simulink model "LUTs"  (Simulink 5.0)
settings: Solver=ode45  StartTime=0.0  StopTime=10.0  RelTol=1e-3
undefined symbols (not defined in the file or in its folder): a_vec, b, Cbar, h_vec, J_FDIR, p_vec, r2d, rho_vec, S, splr_vec, T_vec, weight
libraries: simulink x14
settings Model: LastModifiedBy=Gpapageo

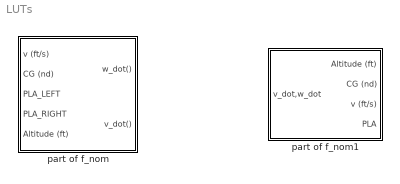
== system LUTs ==
  part of f_nom : Subsystem
  part of f_nom1 : Subsystem  Orientation=left

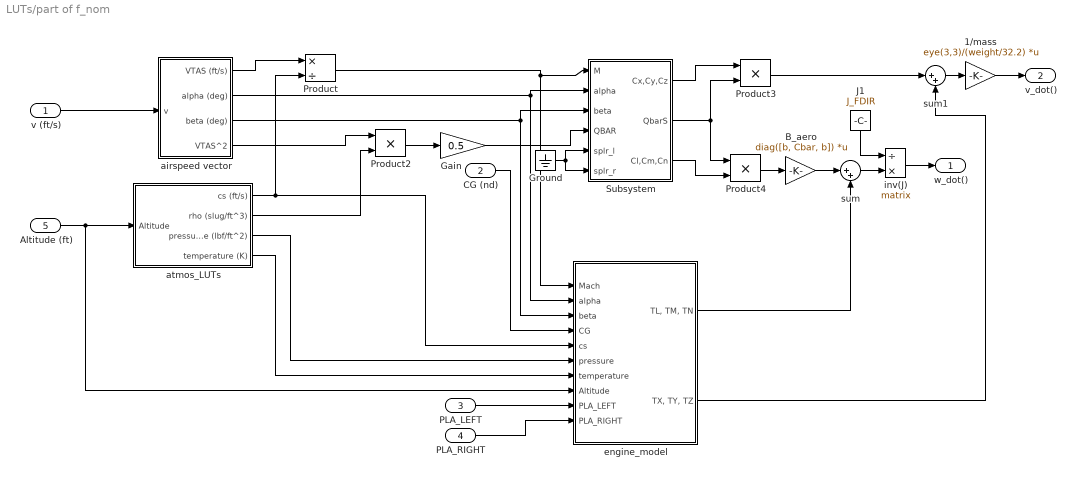
== system LUTs/part of f_nom ==
  v (ft/s) : Inport
  CG (nd) : Inport  Port=2
  PLA_LEFT : Inport  Port=3
  PLA_RIGHT : Inport  Port=4
  Altitude (ft) : Inport  Port=5
  1/mass : Gain  Gain=eye(3,3)/(weight/32.2)  Multiplication=Matrix(K*u)  SaturateOnIntegerOverflow=on
  B_aero : Gain  Gain=diag([b, Cbar, b])  Multiplication=Matrix(K*u)  SaturateOnIntegerOverflow=on
  Gain : Gain  Gain=0.5  SaturateOnIntegerOverflow=on
  Ground : Ground
  J1 : Constant  Orientation=down  Value=J_FDIR
  Product : Product  Inputs=*/  SaturateOnIntegerOverflow=on
  Product2 : Product  SaturateOnIntegerOverflow=on
  Product3 : Product  SaturateOnIntegerOverflow=on
  Product4 : Product  SaturateOnIntegerOverflow=on
  Subsystem : Subsystem
  airspeed vector : Subsystem
  atmos_LUTs : Subsystem
  engine_model : Subsystem
  inv(J) : Product  Inputs=/*  Multiplication=Matrix(*)  SaturateOnIntegerOverflow=on  InputSameDT=on
  sum : Sum  Inputs=|++  InputSameDT=on
  sum1 : Sum  Inputs=|++  InputSameDT=on
  w_dot() : Outport
  v_dot() : Outport  Port=2
  wires:
  sum1/1 -> 1/mass/1
  engine_model/1("TL, TM, TN") -> sum/2
  engine_model/2("TX, TY, TZ") -> sum1/2
  Product3/1 -> sum1/1
  1/mass/1 -> v_dot()/1
  sum/1 -> inv(J)/2
  B_aero/1 -> sum/1
  Subsystem/2(QbarS) -> Product4/1, Product3/2
  Subsystem/3(Cl,Cm,Cn) -> Product4/2
  Subsystem/1(Cx,Cy,Cz) -> Product3/1
  inv(J)/1 -> w_dot()/1
  Product4/1 -> B_aero/1
  J1/1 -> inv(J)/1
  PLA_RIGHT/1 -> engine_model/10(PLA_RIGHT)
  PLA_LEFT/1 -> engine_model/9(PLA_LEFT)
  atmos_LUTs/4(temperature (K)) -> engine_model/7(temperature)
  atmos_LUTs/3(pressure (lbf/ft^2)) -> engine_model/6(pressure)
  atmos_LUTs/1(cs (ft/s)) -> engine_model/5(cs), Product/2
  Product2/1 -> Gain/1
  airspeed vector/4(VTAS^2) -> Product2/1
  CG (nd)/1 -> engine_model/4(CG)
  v (ft/s)/1 -> airspeed vector/1(v)
  Altitude (ft)/1 -> engine_model/8(Altitude), atmos_LUTs/1(Altitude)
  atmos_LUTs/2(rho (slug/ft^3)) -> Product2/2
  airspeed vector/1(VTAS (ft/s)) -> Product/1
  airspeed vector/3(beta (deg)) -> engine_model/3(beta), Subsystem/3(beta)
  airspeed vector/2(alpha (deg)) -> engine_model/2(alpha), Subsystem/2(alpha)
  Product/1 -> engine_model/1(Mach), Subsystem/1(M)
  Gain/1 -> Subsystem/4(QBAR)
  Ground/1 -> Subsystem/5(splr_l), Subsystem/6(splr_r)

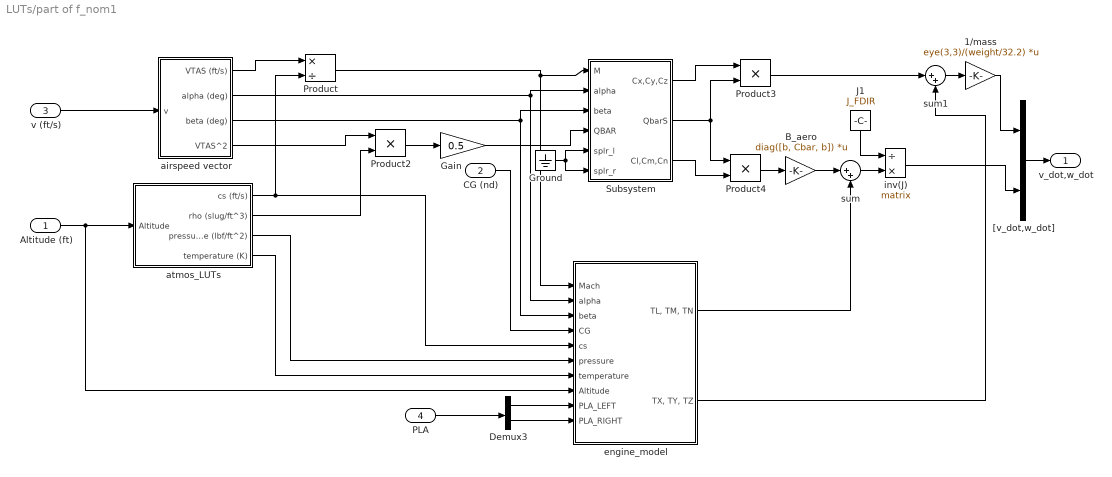
== system LUTs/part of f_nom1 ==
  Altitude (ft) : Inport
  CG (nd) : Inport  Port=2
  v (ft/s) : Inport  Port=3
  PLA : Inport  Port=4
  1/mass : Gain  Gain=eye(3,3)/(weight/32.2)  Multiplication=Matrix(K*u)  SaturateOnIntegerOverflow=on
  B_aero : Gain  Gain=diag([b, Cbar, b])  Multiplication=Matrix(K*u)  SaturateOnIntegerOverflow=on
  Demux3 : Demux  Outputs=2
  Gain : Gain  Gain=0.5  SaturateOnIntegerOverflow=on
  Ground : Ground
  J1 : Constant  Orientation=down  Value=J_FDIR
  Product : Product  Inputs=*/  SaturateOnIntegerOverflow=on
  Product2 : Product  SaturateOnIntegerOverflow=on
  Product3 : Product  SaturateOnIntegerOverflow=on
  Product4 : Product  SaturateOnIntegerOverflow=on
  Subsystem : Subsystem
  "[v_dot,w_dot]" : Mux  Inputs=[3 3]
  airspeed vector : Subsystem
  atmos_LUTs : Subsystem
  engine_model : Subsystem
  inv(J) : Product  Inputs=/*  Multiplication=Matrix(*)  SaturateOnIntegerOverflow=on  InputSameDT=on
  sum : Sum  Inputs=|++  InputSameDT=on
  sum1 : Sum  Inputs=|++  InputSameDT=on
  v_dot,w_dot : Outport
  wires:
  Ground/1 -> Subsystem/6(splr_r), Subsystem/5(splr_l)
  Gain/1 -> Subsystem/4(QBAR)
  Product/1 -> Subsystem/1(M), engine_model/1(Mach)
  airspeed vector/2(alpha (deg)) -> Subsystem/2(alpha), engine_model/2(alpha)
  airspeed vector/3(beta (deg)) -> Subsystem/3(beta), engine_model/3(beta)
  airspeed vector/1(VTAS (ft/s)) -> Product/1
  atmos_LUTs/2(rho (slug/ft^3)) -> Product2/2
  Altitude (ft)/1 -> atmos_LUTs/1(Altitude), engine_model/8(Altitude)
  v (ft/s)/1 -> airspeed vector/1(v)
  CG (nd)/1 -> engine_model/4(CG)
  airspeed vector/4(VTAS^2) -> Product2/1
  Product2/1 -> Gain/1
  atmos_LUTs/1(cs (ft/s)) -> Product/2, engine_model/5(cs)
  atmos_LUTs/3(pressure (lbf/ft^2)) -> engine_model/6(pressure)
  atmos_LUTs/4(temperature (K)) -> engine_model/7(temperature)
  J1/1 -> inv(J)/1
  Product4/1 -> B_aero/1
  Subsystem/1(Cx,Cy,Cz) -> Product3/1
  Subsystem/3(Cl,Cm,Cn) -> Product4/2
  Subsystem/2(QbarS) -> Product3/2, Product4/1
  B_aero/1 -> sum/1
  sum/1 -> inv(J)/2
  Product3/1 -> sum1/1
  engine_model/2("TX, TY, TZ") -> sum1/2
  engine_model/1("TL, TM, TN") -> sum/2
  sum1/1 -> 1/mass/1
  PLA/1 -> Demux3/1
  Demux3/1 -> engine_model/9(PLA_LEFT)
  Demux3/2 -> engine_model/10(PLA_RIGHT)
  inv(J)/1 -> "[v_dot,w_dot]"/2
  "[v_dot,w_dot]"/1 -> v_dot,w_dot/1
  1/mass/1 -> "[v_dot,w_dot]"/1

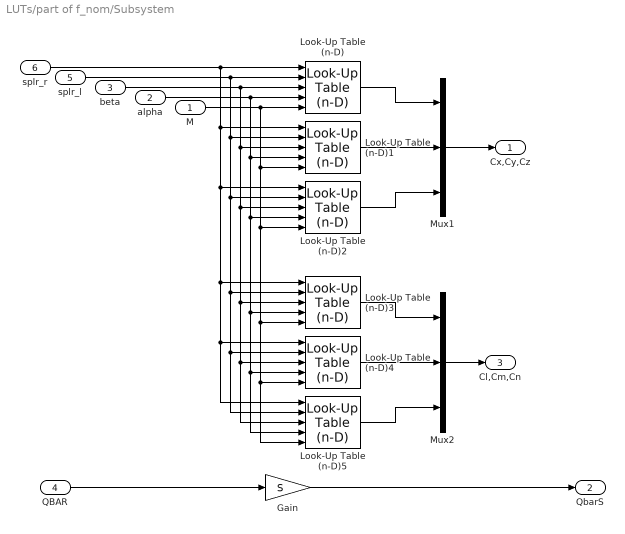
== system LUTs/part of f_nom/Subsystem ==
  M : Inport
  alpha : Inport  Port=2
  beta : Inport  Port=3
  QBAR : Inport  Port=4
  splr_l : Inport  Port=5
  splr_r : Inport  Port=6
  Gain : Gain  Gain=S  SaturateOnIntegerOverflow=on
  Look-Up Table (n-D) : simulink/Look-Up Tables/Look-Up Table (n-D)  numDimsPopupSelect=More...  bp1=splr_vec  bp2=splr_vec  bp3=beta_vec  bp4=alpha_vec  bpcell={M_vec}  explicitNumDims=5  searchMode=Binary Search  cacheBpFlag=on  vectorInputFlag=off  tableData=CX_mat  interpMethod=Linear  extrapMethod=Linear  rangeErrorMode=None
  Look-Up Table (n-D)1 : simulink/Look-Up Tables/Look-Up Table (n-D)  numDimsPopupSelect=More...  bp1=splr_vec  bp2=splr_vec  bp3=beta_vec  bp4=alpha_vec  bpcell={M_vec}  explicitNumDims=5  searchMode=Binary Search  cacheBpFlag=on  vectorInputFlag=off  tableData=CY_mat  interpMethod=Linear  extrapMethod=Linear  rangeErrorMode=None
  Look-Up Table (n-D)2 : simulink/Look-Up Tables/Look-Up Table (n-D)  numDimsPopupSelect=More...  bp1=splr_vec  bp2=splr_vec  bp3=beta_vec  bp4=alpha_vec  bpcell={M_vec}  explicitNumDims=5  searchMode=Binary Search  cacheBpFlag=on  vectorInputFlag=off  tableData=CZ_mat  interpMethod=Linear  extrapMethod=Linear  rangeErrorMode=None
  Look-Up Table (n-D)3 : simulink/Look-Up Tables/Look-Up Table (n-D)  numDimsPopupSelect=More...  bp1=splr_vec  bp2=splr_vec  bp3=beta_vec  bp4=alpha_vec  bpcell={M_vec}  explicitNumDims=5  searchMode=Binary Search  cacheBpFlag=on  vectorInputFlag=off  tableData=CL_mat  interpMethod=Linear  extrapMethod=Linear  rangeErrorMode=None
  Look-Up Table (n-D)4 : simulink/Look-Up Tables/Look-Up Table (n-D)  numDimsPopupSelect=More...  bp1=splr_vec  bp2=splr_vec  bp3=beta_vec  bp4=alpha_vec  bpcell={M_vec}  explicitNumDims=5  searchMode=Binary Search  cacheBpFlag=on  vectorInputFlag=off  tableData=CM_mat  interpMethod=Linear  extrapMethod=Linear  rangeErrorMode=None
  Look-Up Table (n-D)5 : simulink/Look-Up Tables/Look-Up Table (n-D)  numDimsPopupSelect=More...  bp1=splr_vec  bp2=splr_vec  bp3=beta_vec  bp4=alpha_vec  bpcell={M_vec}  explicitNumDims=5  searchMode=Binary Search  cacheBpFlag=on  vectorInputFlag=off  tableData=CN_mat  interpMethod=Linear  extrapMethod=Linear  rangeErrorMode=None
  Mux1 : Mux  Inputs=3
  Mux2 : Mux  Inputs=3
  Cx,Cy,Cz : Outport
  QbarS : Outport  Port=2
  Cl,Cm,Cn : Outport  Port=3
  wires:
  Gain/1 -> QbarS/1
  QBAR/1 -> Gain/1
  Mux2/1 -> Cl,Cm,Cn/1
  Mux1/1 -> Cx,Cy,Cz/1
  splr_r/1 -> Look-Up Table (n-D)/1, Look-Up Table (n-D)1/1, Look-Up Table (n-D)2/1, Look-Up Table (n-D)3/1, Look-Up Table (n-D)4/1, Look-Up Table (n-D)5/1
  splr_l/1 -> Look-Up Table (n-D)/2, Look-Up Table (n-D)1/2, Look-Up Table (n-D)2/2, Look-Up Table (n-D)3/2, Look-Up Table (n-D)4/2, Look-Up Table (n-D)5/2
  beta/1 -> Look-Up Table (n-D)/3, Look-Up Table (n-D)1/3, Look-Up Table (n-D)2/3, Look-Up Table (n-D)3/3, Look-Up Table (n-D)4/3, Look-Up Table (n-D)5/3
  alpha/1 -> Look-Up Table (n-D)/4, Look-Up Table (n-D)1/4, Look-Up Table (n-D)2/4, Look-Up Table (n-D)3/4, Look-Up Table (n-D)4/4, Look-Up Table (n-D)5/4
  M/1 -> Look-Up Table (n-D)/5, Look-Up Table (n-D)1/5, Look-Up Table (n-D)2/5, Look-Up Table (n-D)3/5, Look-Up Table (n-D)4/5, Look-Up Table (n-D)5/5
  Look-Up Table (n-D)/1 -> Mux1/1
  Look-Up Table (n-D)1/1 -> Mux1/2
  Look-Up Table (n-D)2/1 -> Mux1/3
  Look-Up Table (n-D)4/1 -> Mux2/2
  Look-Up Table (n-D)3/1 -> Mux2/1
  Look-Up Table (n-D)5/1 -> Mux2/3

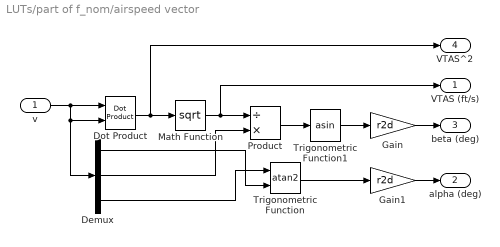
== system LUTs/part of f_nom/airspeed vector ==
  v : Inport  PortDimensions=3
  Demux : Demux  Outputs=3
  Dot Product : simulink/Math Operations/Dot Product
  Gain : Gain  Gain=r2d  SaturateOnIntegerOverflow=on
  Gain1 : Gain  Gain=r2d  SaturateOnIntegerOverflow=on
  Math Function : Math  Operator=sqrt
  Product : Product  Inputs=/*  SaturateOnIntegerOverflow=on  InputSameDT=on
  Trigonometric Function : Trigonometry  Operator=atan2
  Trigonometric Function1 : Trigonometry  Operator=asin
  VTAS (ft/s) : Outport
  alpha (deg) : Outport  Port=2
  beta (deg) : Outport  Port=3
  VTAS^2 : Outport  Port=4
  wires:
  Gain1/1 -> alpha (deg)/1
  Gain/1 -> beta (deg)/1
  Demux/3 -> Trigonometric Function/1
  Demux/1 -> Trigonometric Function/2
  v/1 -> Dot Product/2, Demux/1, Dot Product/1
  Dot Product/1 -> VTAS^2/1, Math Function/1
  Demux/2 -> Product/2
  Product/1 -> Trigonometric Function1/1
  Math Function/1 -> Product/1, VTAS (ft/s)/1
  Trigonometric Function1/1 -> Gain/1
  Trigonometric Function/1 -> Gain1/1

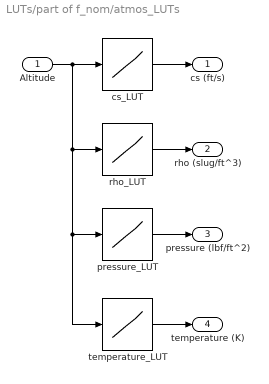
== system LUTs/part of f_nom/atmos_LUTs ==
  Altitude : Inport
  cs_LUT : Lookup  InputValues=h_vec  OutputValues=a_vec  SaturateOnIntegerOverflow=on
  pressure_LUT : Lookup  InputValues=h_vec  OutputValues=p_vec  SaturateOnIntegerOverflow=on
  rho_LUT : Lookup  InputValues=h_vec  OutputValues=rho_vec  SaturateOnIntegerOverflow=on
  temperature_LUT : Lookup  InputValues=h_vec  OutputValues=T_vec  SaturateOnIntegerOverflow=on
  cs (ft/s) : Outport
  rho (slug/ft^3) : Outport  Port=2
  pressure (lbf/ft^2) : Outport  Port=3
  temperature (K) : Outport  Port=4
  wires:
  temperature_LUT/1 -> temperature (K)/1
  pressure_LUT/1 -> pressure (lbf/ft^2)/1
  rho_LUT/1 -> rho (slug/ft^3)/1
  cs_LUT/1 -> cs (ft/s)/1
  Altitude/1 -> pressure_LUT/1, temperature_LUT/1, rho_LUT/1, cs_LUT/1

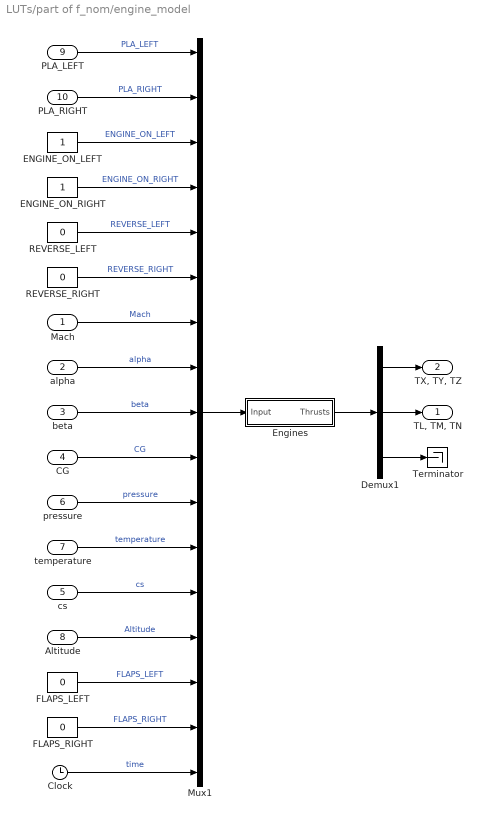
== system LUTs/part of f_nom/engine_model ==
  Mach : Inport
  alpha : Inport  Port=2
  beta : Inport  Port=3
  CG : Inport  Port=4
  cs : Inport  Port=5
  pressure : Inport  Port=6
  temperature : Inport  Port=7
  Altitude : Inport  Port=8
  PLA_LEFT : Inport  Port=9
  PLA_RIGHT : Inport  Port=10
  Clock : Clock
      settings: Decimation=10
  Demux1 : Demux  Outputs=[3 3 5]
  ENGINE_ON_LEFT : Constant
  ENGINE_ON_RIGHT : Constant
  Engines : Subsystem
  FLAPS_LEFT : Constant  Value=0
  FLAPS_RIGHT : Constant  Value=0
  Mux1 : Mux  Inputs=17
  REVERSE_LEFT : Constant  Value=0
  REVERSE_RIGHT : Constant  Value=0
  Terminator : Terminator
  "TL, TM, TN" : Outport
  "TX, TY, TZ" : Outport  Port=2
  wires:
  Clock/1 -> Mux1/17  "time"
  FLAPS_RIGHT/1 -> Mux1/16  "FLAPS_RIGHT"
  Altitude/1 -> Mux1/14  "Altitude"
  FLAPS_LEFT/1 -> Mux1/15  "FLAPS_LEFT"
  cs/1 -> Mux1/13  "cs"
  temperature/1 -> Mux1/12  "temperature"
  pressure/1 -> Mux1/11  "pressure"
  CG/1 -> Mux1/10  "CG"
  beta/1 -> Mux1/9  "beta"
  alpha/1 -> Mux1/8  "alpha"
  Mach/1 -> Mux1/7  "Mach"
  REVERSE_RIGHT/1 -> Mux1/6  "REVERSE_RIGHT"
  REVERSE_LEFT/1 -> Mux1/5  "REVERSE_LEFT"
  ENGINE_ON_RIGHT/1 -> Mux1/4  "ENGINE_ON_RIGHT"
  ENGINE_ON_LEFT/1 -> Mux1/3  "ENGINE_ON_LEFT"
  PLA_RIGHT/1 -> Mux1/2  "PLA_RIGHT"
  PLA_LEFT/1 -> Mux1/1  "PLA_LEFT"
  Engines/1(Thrusts) -> Demux1/1
  Demux1/1 -> "TX, TY, TZ"/1
  Demux1/2 -> "TL, TM, TN"/1
  Demux1/3 -> Terminator/1
  Mux1/1 -> Engines/1(Input)

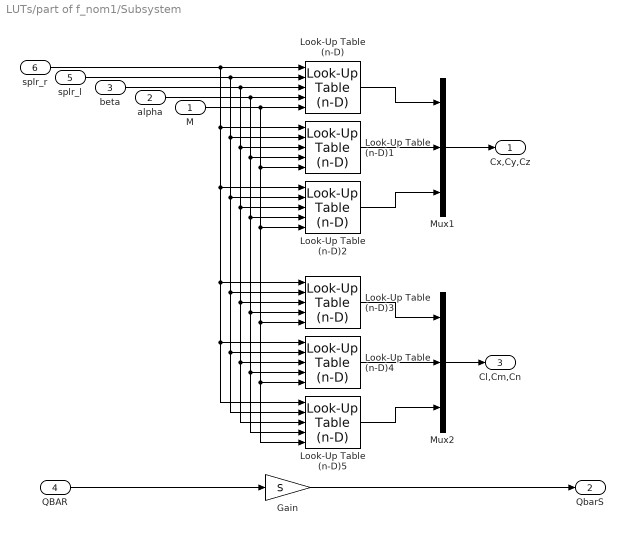
== system LUTs/part of f_nom1/Subsystem ==
  M : Inport
  alpha : Inport  Port=2
  beta : Inport  Port=3
  QBAR : Inport  Port=4
  splr_l : Inport  Port=5
  splr_r : Inport  Port=6
  Gain : Gain  Gain=S  SaturateOnIntegerOverflow=on
  Look-Up Table (n-D) : simulink/Look-Up Tables/Look-Up Table (n-D)  numDimsPopupSelect=More...  bp1=splr_vec  bp2=splr_vec  bp3=beta_vec  bp4=alpha_vec  bpcell={M_vec}  explicitNumDims=5  searchMode=Binary Search  cacheBpFlag=on  vectorInputFlag=off  tableData=CX_mat  interpMethod=Linear  extrapMethod=Linear  rangeErrorMode=None
  Look-Up Table (n-D)1 : simulink/Look-Up Tables/Look-Up Table (n-D)  numDimsPopupSelect=More...  bp1=splr_vec  bp2=splr_vec  bp3=beta_vec  bp4=alpha_vec  bpcell={M_vec}  explicitNumDims=5  searchMode=Binary Search  cacheBpFlag=on  vectorInputFlag=off  tableData=CY_mat  interpMethod=Linear  extrapMethod=Linear  rangeErrorMode=None
  Look-Up Table (n-D)2 : simulink/Look-Up Tables/Look-Up Table (n-D)  numDimsPopupSelect=More...  bp1=splr_vec  bp2=splr_vec  bp3=beta_vec  bp4=alpha_vec  bpcell={M_vec}  explicitNumDims=5  searchMode=Binary Search  cacheBpFlag=on  vectorInputFlag=off  tableData=CZ_mat  interpMethod=Linear  extrapMethod=Linear  rangeErrorMode=None
  Look-Up Table (n-D)3 : simulink/Look-Up Tables/Look-Up Table (n-D)  numDimsPopupSelect=More...  bp1=splr_vec  bp2=splr_vec  bp3=beta_vec  bp4=alpha_vec  bpcell={M_vec}  explicitNumDims=5  searchMode=Binary Search  cacheBpFlag=on  vectorInputFlag=off  tableData=CL_mat  interpMethod=Linear  extrapMethod=Linear  rangeErrorMode=None
  Look-Up Table (n-D)4 : simulink/Look-Up Tables/Look-Up Table (n-D)  numDimsPopupSelect=More...  bp1=splr_vec  bp2=splr_vec  bp3=beta_vec  bp4=alpha_vec  bpcell={M_vec}  explicitNumDims=5  searchMode=Binary Search  cacheBpFlag=on  vectorInputFlag=off  tableData=CM_mat  interpMethod=Linear  extrapMethod=Linear  rangeErrorMode=None
  Look-Up Table (n-D)5 : simulink/Look-Up Tables/Look-Up Table (n-D)  numDimsPopupSelect=More...  bp1=splr_vec  bp2=splr_vec  bp3=beta_vec  bp4=alpha_vec  bpcell={M_vec}  explicitNumDims=5  searchMode=Binary Search  cacheBpFlag=on  vectorInputFlag=off  tableData=CN_mat  interpMethod=Linear  extrapMethod=Linear  rangeErrorMode=None
  Mux1 : Mux  Inputs=3
  Mux2 : Mux  Inputs=3
  Cx,Cy,Cz : Outport
  QbarS : Outport  Port=2
  Cl,Cm,Cn : Outport  Port=3
  wires:
  Look-Up Table (n-D)5/1 -> Mux2/3
  Look-Up Table (n-D)3/1 -> Mux2/1
  Look-Up Table (n-D)4/1 -> Mux2/2
  Look-Up Table (n-D)2/1 -> Mux1/3
  Look-Up Table (n-D)1/1 -> Mux1/2
  Look-Up Table (n-D)/1 -> Mux1/1
  M/1 -> Look-Up Table (n-D)5/5, Look-Up Table (n-D)4/5, Look-Up Table (n-D)3/5, Look-Up Table (n-D)2/5, Look-Up Table (n-D)1/5, Look-Up Table (n-D)/5
  alpha/1 -> Look-Up Table (n-D)5/4, Look-Up Table (n-D)4/4, Look-Up Table (n-D)3/4, Look-Up Table (n-D)2/4, Look-Up Table (n-D)1/4, Look-Up Table (n-D)/4
  beta/1 -> Look-Up Table (n-D)5/3, Look-Up Table (n-D)4/3, Look-Up Table (n-D)3/3, Look-Up Table (n-D)2/3, Look-Up Table (n-D)1/3, Look-Up Table (n-D)/3
  splr_l/1 -> Look-Up Table (n-D)5/2, Look-Up Table (n-D)4/2, Look-Up Table (n-D)3/2, Look-Up Table (n-D)2/2, Look-Up Table (n-D)1/2, Look-Up Table (n-D)/2
  splr_r/1 -> Look-Up Table (n-D)5/1, Look-Up Table (n-D)4/1, Look-Up Table (n-D)3/1, Look-Up Table (n-D)2/1, Look-Up Table (n-D)1/1, Look-Up Table (n-D)/1
  Mux1/1 -> Cx,Cy,Cz/1
  Mux2/1 -> Cl,Cm,Cn/1
  QBAR/1 -> Gain/1
  Gain/1 -> QbarS/1

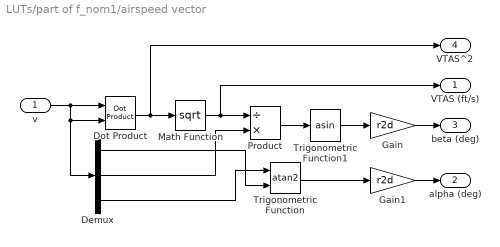
== system LUTs/part of f_nom1/airspeed vector ==
  v : Inport  PortDimensions=3
  Demux : Demux  Outputs=3
  Dot Product : simulink/Math Operations/Dot Product
  Gain : Gain  Gain=r2d  SaturateOnIntegerOverflow=on
  Gain1 : Gain  Gain=r2d  SaturateOnIntegerOverflow=on
  Math Function : Math  Operator=sqrt
  Product : Product  Inputs=/*  SaturateOnIntegerOverflow=on  InputSameDT=on
  Trigonometric Function : Trigonometry  Operator=atan2
  Trigonometric Function1 : Trigonometry  Operator=asin
  VTAS (ft/s) : Outport
  alpha (deg) : Outport  Port=2
  beta (deg) : Outport  Port=3
  VTAS^2 : Outport  Port=4
  wires:
  Trigonometric Function/1 -> Gain1/1
  Trigonometric Function1/1 -> Gain/1
  Math Function/1 -> VTAS (ft/s)/1, Product/1
  Product/1 -> Trigonometric Function1/1
  Demux/2 -> Product/2
  Dot Product/1 -> Math Function/1, VTAS^2/1
  v/1 -> Dot Product/1, Demux/1, Dot Product/2
  Demux/1 -> Trigonometric Function/2
  Demux/3 -> Trigonometric Function/1
  Gain/1 -> beta (deg)/1
  Gain1/1 -> alpha (deg)/1

== system LUTs/part of f_nom1/atmos_LUTs ==
  Altitude : Inport
  cs_LUT : Lookup  InputValues=h_vec  OutputValues=a_vec  SaturateOnIntegerOverflow=on
  pressure_LUT : Lookup  InputValues=h_vec  OutputValues=p_vec  SaturateOnIntegerOverflow=on
  rho_LUT : Lookup  InputValues=h_vec  OutputValues=rho_vec  SaturateOnIntegerOverflow=on
  temperature_LUT : Lookup  InputValues=h_vec  OutputValues=T_vec  SaturateOnIntegerOverflow=on
  cs (ft/s) : Outport
  rho (slug/ft^3) : Outport  Port=2
  pressure (lbf/ft^2) : Outport  Port=3
  temperature (K) : Outport  Port=4
  wires:
  Altitude/1 -> cs_LUT/1, rho_LUT/1, temperature_LUT/1, pressure_LUT/1
  cs_LUT/1 -> cs (ft/s)/1
  rho_LUT/1 -> rho (slug/ft^3)/1
  pressure_LUT/1 -> pressure (lbf/ft^2)/1
  temperature_LUT/1 -> temperature (K)/1

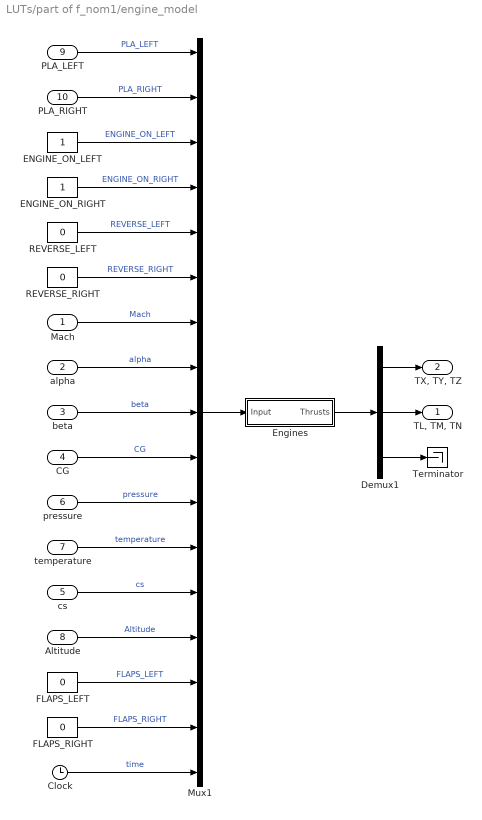
== system LUTs/part of f_nom1/engine_model ==
  Mach : Inport
  alpha : Inport  Port=2
  beta : Inport  Port=3
  CG : Inport  Port=4
  cs : Inport  Port=5
  pressure : Inport  Port=6
  temperature : Inport  Port=7
  Altitude : Inport  Port=8
  PLA_LEFT : Inport  Port=9
  PLA_RIGHT : Inport  Port=10
  Clock : Clock
      settings: Decimation=10
  Demux1 : Demux  Outputs=[3 3 5]
  ENGINE_ON_LEFT : Constant
  ENGINE_ON_RIGHT : Constant
  Engines : Subsystem
  FLAPS_LEFT : Constant  Value=0
  FLAPS_RIGHT : Constant  Value=0
  Mux1 : Mux  Inputs=17
  REVERSE_LEFT : Constant  Value=0
  REVERSE_RIGHT : Constant  Value=0
  Terminator : Terminator
  "TL, TM, TN" : Outport
  "TX, TY, TZ" : Outport  Port=2
  wires:
  Mux1/1 -> Engines/1(Input)
  Demux1/3 -> Terminator/1
  Demux1/2 -> "TL, TM, TN"/1
  Demux1/1 -> "TX, TY, TZ"/1
  Engines/1(Thrusts) -> Demux1/1
  PLA_LEFT/1 -> Mux1/1  "PLA_LEFT"
  PLA_RIGHT/1 -> Mux1/2  "PLA_RIGHT"
  ENGINE_ON_LEFT/1 -> Mux1/3  "ENGINE_ON_LEFT"
  ENGINE_ON_RIGHT/1 -> Mux1/4  "ENGINE_ON_RIGHT"
  REVERSE_LEFT/1 -> Mux1/5  "REVERSE_LEFT"
  REVERSE_RIGHT/1 -> Mux1/6  "REVERSE_RIGHT"
  Mach/1 -> Mux1/7  "Mach"
  alpha/1 -> Mux1/8  "alpha"
  beta/1 -> Mux1/9  "beta"
  CG/1 -> Mux1/10  "CG"
  pressure/1 -> Mux1/11  "pressure"
  temperature/1 -> Mux1/12  "temperature"
  cs/1 -> Mux1/13  "cs"
  FLAPS_LEFT/1 -> Mux1/15  "FLAPS_LEFT"
  Altitude/1 -> Mux1/14  "Altitude"
  FLAPS_RIGHT/1 -> Mux1/16  "FLAPS_RIGHT"
  Clock/1 -> Mux1/17  "time"

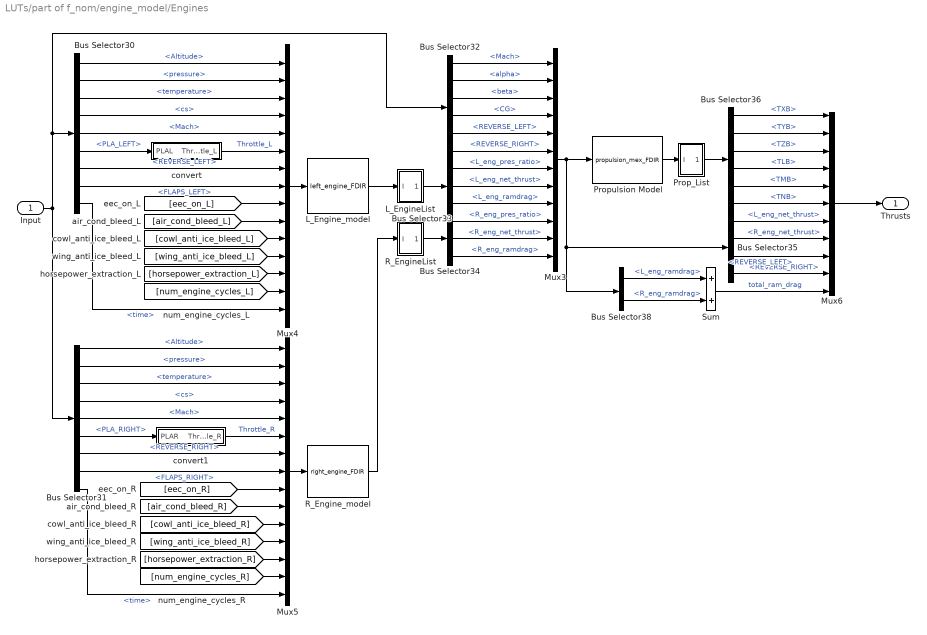
== system LUTs/part of f_nom/engine_model/Engines ==
  Input : Inport
  Bus Selector30 : BusSelector  OutputSignals=Altitude,pressure,temperature,cs,Mach,PLA_LEFT,REVERSE_LEFT,FLAPS_LEFT,time
  Bus Selector31 : BusSelector  OutputSignals=Altitude,pressure,temperature,cs,Mach,PLA_RIGHT,REVERSE_RIGHT,FLAPS_RIGHT,time
  Bus Selector32 : BusSelector  OutputSignals=Mach,alpha,beta,CG,REVERSE_LEFT,REVERSE_RIGHT
  Bus Selector33 : BusSelector  OutputSignals=L_eng_pres_ratio,L_eng_net_thrust,L_eng_ramdrag
  Bus Selector34 : BusSelector  OutputSignals=R_eng_pres_ratio,R_eng_net_thrust,R_eng_ramdrag
  Bus Selector35 : BusSelector  OutputSignals=L_eng_net_thrust,R_eng_net_thrust,REVERSE_LEFT,REVERSE_RIGHT
  Bus Selector36 : BusSelector  OutputSignals=TXB,TYB,TZB,TLB,TMB,TNB
  Bus Selector38 : BusSelector  OutputSignals=L_eng_ramdrag,R_eng_ramdrag
  L_EngineList : Subsystem
  L_Engine_model : S-Function  FunctionName=left_engine_FDIR
  Mux3 : Mux  Inputs=12
  Mux4 : Mux  Inputs=15
  Mux5 : Mux  Inputs=15
  Mux6 : Mux  Inputs=11
  Prop_List : Subsystem
  Propulsion Model : S-Function  FunctionName=propulsion_mex_FDIR
  R_EngineList : Subsystem
  R_Engine_model : S-Function  FunctionName=right_engine_FDIR
  Sum : Sum  SaturateOnIntegerOverflow=on  InputSameDT=on
  convert : Subsystem
  convert1 : Subsystem
  Thrusts : Outport
  wires:
  R_EngineList/1(O) -> Bus Selector34/1
  L_EngineList/1(O) -> Bus Selector33/1
  Mux6/1 -> Thrusts/1
  [horsepower_extraction_R] -> Mux5/13
  [cowl_anti_ice_bleed_R] -> Mux5/11
  Mux4/1 -> L_Engine_model/1
  Mux5/1 -> R_Engine_model/1
  [num_engine_cycles_R] -> Mux5/14
  [wing_anti_ice_bleed_R] -> Mux5/12
  [air_cond_bleed_R] -> Mux5/10
  [eec_on_R] -> Mux5/9
  Bus Selector31/9 -> Mux5/15  "<time>"
  Bus Selector31/4 -> Mux5/4  "<cs>"
  convert1/1(Throttle_R) -> Mux5/6  "Throttle_R"
  Bus Selector31/6 -> convert1/1(PLAR)  "<PLA_RIGHT>"
  Bus Selector31/8 -> Mux5/8  "<FLAPS_RIGHT>"
  Bus Selector31/7 -> Mux5/7  "<REVERSE_RIGHT>"
  Bus Selector31/5 -> Mux5/5  "<Mach>"
  Bus Selector31/3 -> Mux5/3  "<temperature>"
  Bus Selector31/2 -> Mux5/2  "<pressure>"
  Bus Selector31/1 -> Mux5/1  "<Altitude>"
  [num_engine_cycles_L] -> Mux4/14
  [horsepower_extraction_L] -> Mux4/13
  [wing_anti_ice_bleed_L] -> Mux4/12
  [cowl_anti_ice_bleed_L] -> Mux4/11
  [air_cond_bleed_L] -> Mux4/10
  [eec_on_L] -> Mux4/9
  Bus Selector30/9 -> Mux4/15  "<time>"
  Bus Selector30/4 -> Mux4/4  "<cs>"
  convert/1(Throttle_L) -> Mux4/6  "Throttle_L"
  Bus Selector30/6 -> convert/1(PLAL)  "<PLA_LEFT>"
  Bus Selector30/8 -> Mux4/8  "<FLAPS_LEFT>"
  Bus Selector30/7 -> Mux4/7  "<REVERSE_LEFT>"
  Bus Selector30/5 -> Mux4/5  "<Mach>"
  Bus Selector30/3 -> Mux4/3  "<temperature>"
  Bus Selector30/2 -> Mux4/2  "<pressure>"
  Bus Selector30/1 -> Mux4/1  "<Altitude>"
  Propulsion Model/1 -> Prop_List/1(I)
  Bus Selector35/4 -> Mux6/10  "<REVERSE_RIGHT>"
  Bus Selector35/3 -> Mux6/9  "<REVERSE_LEFT>"
  Bus Selector35/2 -> Mux6/8  "<R_eng_net_thrust>"
  Bus Selector35/1 -> Mux6/7  "<L_eng_net_thrust>"
  Bus Selector36/6 -> Mux6/6  "<TNB>"
  Bus Selector36/5 -> Mux6/5  "<TMB>"
  Bus Selector36/4 -> Mux6/4  "<TLB>"
  Bus Selector36/2 -> Mux6/2  "<TYB>"
  Bus Selector36/3 -> Mux6/3  "<TZB>"
  Bus Selector36/1 -> Mux6/1  "<TXB>"
  Bus Selector38/2 -> Sum/2  "<R_eng_ramdrag>"
  Bus Selector38/1 -> Sum/1  "<L_eng_ramdrag>"
  Sum/1 -> Mux6/11  "total_ram_drag"
  Prop_List/1(O) -> Bus Selector36/1
  Mux3/1 -> Bus Selector38/1, Bus Selector35/1, Propulsion Model/1
  Bus Selector34/3 -> Mux3/12  "<R_eng_ramdrag>"
  Bus Selector34/2 -> Mux3/11  "<R_eng_net_thrust>"
  Bus Selector34/1 -> Mux3/10  "<R_eng_pres_ratio>"
  Bus Selector33/3 -> Mux3/9  "<L_eng_ramdrag>"
  Bus Selector33/2 -> Mux3/8  "<L_eng_net_thrust>"
  Bus Selector33/1 -> Mux3/7  "<L_eng_pres_ratio>"
  Bus Selector32/6 -> Mux3/6  "<REVERSE_RIGHT>"
  Bus Selector32/5 -> Mux3/5  "<REVERSE_LEFT>"
  Bus Selector32/4 -> Mux3/4  "<CG>"
  Bus Selector32/3 -> Mux3/3  "<beta>"
  Bus Selector32/2 -> Mux3/2  "<alpha>"
  Bus Selector32/1 -> Mux3/1  "<Mach>"
  R_Engine_model/1 -> R_EngineList/1(I)
  L_Engine_model/1 -> L_EngineList/1(I)
  Input/1 -> Bus Selector30/1, Bus Selector32/1, Bus Selector31/1

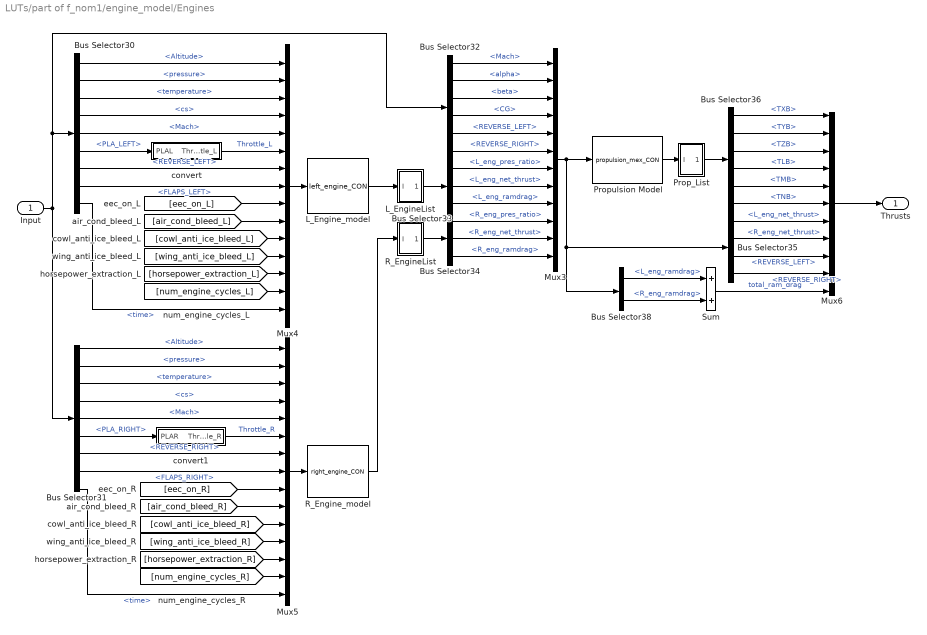
== system LUTs/part of f_nom1/engine_model/Engines ==
  Input : Inport
  Bus Selector30 : BusSelector  OutputSignals=Altitude,pressure,temperature,cs,Mach,PLA_LEFT,REVERSE_LEFT,FLAPS_LEFT,time
  Bus Selector31 : BusSelector  OutputSignals=Altitude,pressure,temperature,cs,Mach,PLA_RIGHT,REVERSE_RIGHT,FLAPS_RIGHT,time
  Bus Selector32 : BusSelector  OutputSignals=Mach,alpha,beta,CG,REVERSE_LEFT,REVERSE_RIGHT
  Bus Selector33 : BusSelector  OutputSignals=L_eng_pres_ratio,L_eng_net_thrust,L_eng_ramdrag
  Bus Selector34 : BusSelector  OutputSignals=R_eng_pres_ratio,R_eng_net_thrust,R_eng_ramdrag
  Bus Selector35 : BusSelector  OutputSignals=L_eng_net_thrust,R_eng_net_thrust,REVERSE_LEFT,REVERSE_RIGHT
  Bus Selector36 : BusSelector  OutputSignals=TXB,TYB,TZB,TLB,TMB,TNB
  Bus Selector38 : BusSelector  OutputSignals=L_eng_ramdrag,R_eng_ramdrag
  L_EngineList : Subsystem
  L_Engine_model : S-Function  FunctionName=left_engine_CON
  Mux3 : Mux  Inputs=12
  Mux4 : Mux  Inputs=15
  Mux5 : Mux  Inputs=15
  Mux6 : Mux  Inputs=11
  Prop_List : Subsystem
  Propulsion Model : S-Function  FunctionName=propulsion_mex_CON
  R_EngineList : Subsystem
  R_Engine_model : S-Function  FunctionName=right_engine_CON
  Sum : Sum  SaturateOnIntegerOverflow=on  InputSameDT=on
  convert : Subsystem
  convert1 : Subsystem
  Thrusts : Outport
  wires:
  Input/1 -> Bus Selector31/1, Bus Selector32/1, Bus Selector30/1
  L_Engine_model/1 -> L_EngineList/1(I)
  R_Engine_model/1 -> R_EngineList/1(I)
  Bus Selector32/1 -> Mux3/1  "<Mach>"
  Bus Selector32/2 -> Mux3/2  "<alpha>"
  Bus Selector32/3 -> Mux3/3  "<beta>"
  Bus Selector32/4 -> Mux3/4  "<CG>"
  Bus Selector32/5 -> Mux3/5  "<REVERSE_LEFT>"
  Bus Selector32/6 -> Mux3/6  "<REVERSE_RIGHT>"
  Bus Selector33/1 -> Mux3/7  "<L_eng_pres_ratio>"
  Bus Selector33/2 -> Mux3/8  "<L_eng_net_thrust>"
  Bus Selector33/3 -> Mux3/9  "<L_eng_ramdrag>"
  Bus Selector34/1 -> Mux3/10  "<R_eng_pres_ratio>"
  Bus Selector34/2 -> Mux3/11  "<R_eng_net_thrust>"
  Bus Selector34/3 -> Mux3/12  "<R_eng_ramdrag>"
  Mux3/1 -> Propulsion Model/1, Bus Selector35/1, Bus Selector38/1
  Prop_List/1(O) -> Bus Selector36/1
  Sum/1 -> Mux6/11  "total_ram_drag"
  Bus Selector38/1 -> Sum/1  "<L_eng_ramdrag>"
  Bus Selector38/2 -> Sum/2  "<R_eng_ramdrag>"
  Bus Selector36/1 -> Mux6/1  "<TXB>"
  Bus Selector36/3 -> Mux6/3  "<TZB>"
  Bus Selector36/2 -> Mux6/2  "<TYB>"
  Bus Selector36/4 -> Mux6/4  "<TLB>"
  Bus Selector36/5 -> Mux6/5  "<TMB>"
  Bus Selector36/6 -> Mux6/6  "<TNB>"
  Bus Selector35/1 -> Mux6/7  "<L_eng_net_thrust>"
  Bus Selector35/2 -> Mux6/8  "<R_eng_net_thrust>"
  Bus Selector35/3 -> Mux6/9  "<REVERSE_LEFT>"
  Bus Selector35/4 -> Mux6/10  "<REVERSE_RIGHT>"
  Propulsion Model/1 -> Prop_List/1(I)
  Bus Selector30/1 -> Mux4/1  "<Altitude>"
  Bus Selector30/2 -> Mux4/2  "<pressure>"
  Bus Selector30/3 -> Mux4/3  "<temperature>"
  Bus Selector30/5 -> Mux4/5  "<Mach>"
  Bus Selector30/7 -> Mux4/7  "<REVERSE_LEFT>"
  Bus Selector30/8 -> Mux4/8  "<FLAPS_LEFT>"
  Bus Selector30/6 -> convert/1(PLAL)  "<PLA_LEFT>"
  convert/1(Throttle_L) -> Mux4/6  "Throttle_L"
  Bus Selector30/4 -> Mux4/4  "<cs>"
  Bus Selector30/9 -> Mux4/15  "<time>"
  [eec_on_L] -> Mux4/9
  [air_cond_bleed_L] -> Mux4/10
  [cowl_anti_ice_bleed_L] -> Mux4/11
  [wing_anti_ice_bleed_L] -> Mux4/12
  [horsepower_extraction_L] -> Mux4/13
  [num_engine_cycles_L] -> Mux4/14
  Bus Selector31/1 -> Mux5/1  "<Altitude>"
  Bus Selector31/2 -> Mux5/2  "<pressure>"
  Bus Selector31/3 -> Mux5/3  "<temperature>"
  Bus Selector31/5 -> Mux5/5  "<Mach>"
  Bus Selector31/7 -> Mux5/7  "<REVERSE_RIGHT>"
  Bus Selector31/8 -> Mux5/8  "<FLAPS_RIGHT>"
  Bus Selector31/6 -> convert1/1(PLAR)  "<PLA_RIGHT>"
  convert1/1(Throttle_R) -> Mux5/6  "Throttle_R"
  Bus Selector31/4 -> Mux5/4  "<cs>"
  Bus Selector31/9 -> Mux5/15  "<time>"
  [eec_on_R] -> Mux5/9
  [air_cond_bleed_R] -> Mux5/10
  [wing_anti_ice_bleed_R] -> Mux5/12
  [num_engine_cycles_R] -> Mux5/14
  Mux5/1 -> R_Engine_model/1
  Mux4/1 -> L_Engine_model/1
  [cowl_anti_ice_bleed_R] -> Mux5/11
  [horsepower_extraction_R] -> Mux5/13
  Mux6/1 -> Thrusts/1
  L_EngineList/1(O) -> Bus Selector33/1
  R_EngineList/1(O) -> Bus Selector34/1

== system LUTs/part of f_nom/engine_model/Engines/L_EngineList ==
  I : Inport
  Demux : Demux  Outputs=6
  Mux : Mux  Inputs=6
  O : Outport
  wires:
  Demux/1 -> Mux/1  "L_eng_net_thrust"
  Demux/6 -> Mux/6  "L_eng_N3"
  Demux/5 -> Mux/5  "L_eng_N2"
  Demux/4 -> Mux/4  "L_eng_N1"
  Demux/3 -> Mux/3  "L_eng_ramdrag"
  Mux/1 -> O/1
  I/1 -> Demux/1
  Demux/2 -> Mux/2  "L_eng_pres_ratio"

== system LUTs/part of f_nom/engine_model/Engines/Prop_List ==
  I : Inport
  Demux : Demux  Outputs=8
  Mux : Mux  Inputs=8
  O : Outport
  wires:
  I/1 -> Demux/1
  Mux/1 -> O/1
  Demux/2 -> Mux/2  "RAM_DRAG_TOTAL"
  Demux/1 -> Mux/1  "THRUST_TOTAL"
  Demux/3 -> Mux/3  "TXB"
  Demux/4 -> Mux/4  "TYB"
  Demux/5 -> Mux/5  "TZB"
  Demux/6 -> Mux/6  "TLB"
  Demux/7 -> Mux/7  "TMB"
  Demux/8 -> Mux/8  "TNB"

== system LUTs/part of f_nom/engine_model/Engines/R_EngineList ==
  I : Inport
  Demux : Demux  Outputs=6
  Mux : Mux  Inputs=6
  O : Outport
  wires:
  Demux/1 -> Mux/1  "R_eng_net_thrust"
  Demux/6 -> Mux/6  "R_eng_N3"
  Demux/5 -> Mux/5  "R_eng_N2"
  Demux/4 -> Mux/4  "R_eng_N1"
  Demux/3 -> Mux/3  "R_eng_ramdrag"
  Mux/1 -> O/1
  I/1 -> Demux/1
  Demux/2 -> Mux/2  "R_eng_pres_ratio"

== system LUTs/part of f_nom/engine_model/Engines/convert ==
  PLAL : Inport
  1/PLA_max-PLA_min : Constant  Value=1/75
  PLA_min : Constant  Value=55.0
  Product : Product  SaturateOnIntegerOverflow=on  InputSameDT=on
  Sum : Sum  Inputs=|+-  SaturateOnIntegerOverflow=on  InputSameDT=on
  Throttle_L : Outport
  wires:
  PLAL/1 -> Sum/1
  Product/1 -> Throttle_L/1  "Throttle_L"
  1/PLA_max-PLA_min/1 -> Product/1
  Sum/1 -> Product/2
  PLA_min/1 -> Sum/2

== system LUTs/part of f_nom/engine_model/Engines/convert1 ==
  PLAR : Inport
  1/PLA_max-PLA_min : Constant  Value=1/75
  PLA_min : Constant  Value=55.0
  Product : Product  SaturateOnIntegerOverflow=on  InputSameDT=on
  Sum : Sum  Inputs=|+-  SaturateOnIntegerOverflow=on  InputSameDT=on
  Throttle_R : Outport
  wires:
  PLAR/1 -> Sum/1
  Product/1 -> Throttle_R/1  "Throttle_R"
  1/PLA_max-PLA_min/1 -> Product/1
  Sum/1 -> Product/2
  PLA_min/1 -> Sum/2

== system LUTs/part of f_nom1/engine_model/Engines/L_EngineList ==
  I : Inport
  Demux : Demux  Outputs=6
  Mux : Mux  Inputs=6
  O : Outport
  wires:
  Demux/2 -> Mux/2  "L_eng_pres_ratio"
  I/1 -> Demux/1
  Mux/1 -> O/1
  Demux/3 -> Mux/3  "L_eng_ramdrag"
  Demux/4 -> Mux/4  "L_eng_N1"
  Demux/5 -> Mux/5  "L_eng_N2"
  Demux/6 -> Mux/6  "L_eng_N3"
  Demux/1 -> Mux/1  "L_eng_net_thrust"

== system LUTs/part of f_nom1/engine_model/Engines/Prop_List ==
  I : Inport
  Demux : Demux  Outputs=8
  Mux : Mux  Inputs=8
  O : Outport
  wires:
  Demux/8 -> Mux/8  "TNB"
  Demux/7 -> Mux/7  "TMB"
  Demux/6 -> Mux/6  "TLB"
  Demux/5 -> Mux/5  "TZB"
  Demux/4 -> Mux/4  "TYB"
  Demux/3 -> Mux/3  "TXB"
  Demux/1 -> Mux/1  "THRUST_TOTAL"
  Demux/2 -> Mux/2  "RAM_DRAG_TOTAL"
  Mux/1 -> O/1
  I/1 -> Demux/1

== system LUTs/part of f_nom1/engine_model/Engines/R_EngineList ==
  I : Inport
  Demux : Demux  Outputs=6
  Mux : Mux  Inputs=6
  O : Outport
  wires:
  Demux/2 -> Mux/2  "R_eng_pres_ratio"
  I/1 -> Demux/1
  Mux/1 -> O/1
  Demux/3 -> Mux/3  "R_eng_ramdrag"
  Demux/4 -> Mux/4  "R_eng_N1"
  Demux/5 -> Mux/5  "R_eng_N2"
  Demux/6 -> Mux/6  "R_eng_N3"
  Demux/1 -> Mux/1  "R_eng_net_thrust"

== system LUTs/part of f_nom1/engine_model/Engines/convert ==
  PLAL : Inport
  1/PLA_max-PLA_min : Constant  Value=1/75
  PLA_min : Constant  Value=55.0
  Product : Product  SaturateOnIntegerOverflow=on  InputSameDT=on
  Sum : Sum  Inputs=|+-  SaturateOnIntegerOverflow=on  InputSameDT=on
  Throttle_L : Outport
  wires:
  PLA_min/1 -> Sum/2
  Sum/1 -> Product/2
  1/PLA_max-PLA_min/1 -> Product/1
  Product/1 -> Throttle_L/1  "Throttle_L"
  PLAL/1 -> Sum/1

== system LUTs/part of f_nom1/engine_model/Engines/convert1 ==
  PLAR : Inport
  1/PLA_max-PLA_min : Constant  Value=1/75
  PLA_min : Constant  Value=55.0
  Product : Product  SaturateOnIntegerOverflow=on  InputSameDT=on
  Sum : Sum  Inputs=|+-  SaturateOnIntegerOverflow=on  InputSameDT=on
  Throttle_R : Outport
  wires:
  PLA_min/1 -> Sum/2
  Sum/1 -> Product/2
  1/PLA_max-PLA_min/1 -> Product/1
  Product/1 -> Throttle_R/1  "Throttle_R"
  PLAR/1 -> Sum/1
